simulink model "PP_hinhhoc"  (R2024a)
settings: Solver=ode4  StartTime=0.0  StopTime=10  FixedStep=0.01  RelTol=1e-3
settings Model: Creator=thunguyen  LastModifiedBy=thunguyen

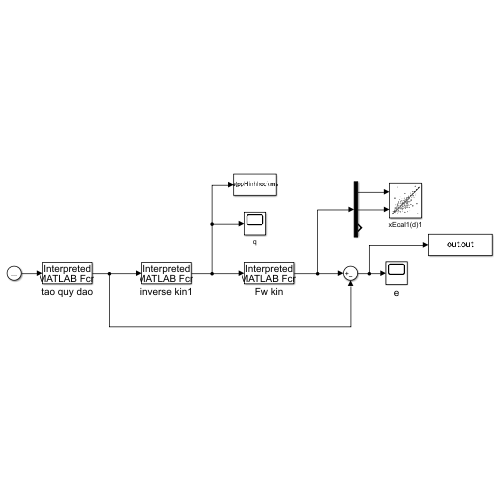
[thumbnail: Simulink's stored preview of the top-level diagram]
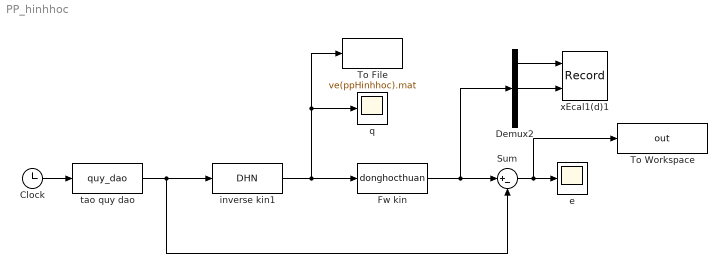
== system PP_hinhhoc ==
  Clock : Clock
  Demux2 : Demux  Outputs=3
  Fw kin : MATLABFcn  MATLABFcn=donghocthuan  OutputDimensions=3  Output1D=off
  Sum : Sum  Inputs=|+-
  To File : ToFile  Filename=ve(ppHinhhoc).mat
  To Workspace : ToWorkspace  VariableName=out  SaveFormat=Timeseries  SampleTime=-1
  e : Scope
  inverse kin1 : MATLABFcn  MATLABFcn=DHN  OutputDimensions=3  Output1D=off
  q : Scope
  tao quy dao : MATLABFcn  MATLABFcn=quy_dao  OutputDimensions=3  Output1D=off
  xEcal1(d)1 : Record  FileSettingsInternal="{\"entries\":[{\"content\":{\"excelSettings\":{\"content\":{},\"type\":\"Streamout.ExcelSettings\"}},\"type\":\"Streamout.FileSettingStorage\",\"uuid\":\"\"}],\"packageUris\":[\"http:\\/\\/schema.mathworks.com\\/mf0\\/streamout_blocks\\/R2020a\"],\"version\":\"1.0\"}"  Layout=[1 1]  SignalsInternal="{\"entries\":[{\"content\":{\"signals\":[{\"content\":{\"blockPath\":[],\"dimensions\":[1],\"domain\":\"\",\"lineColor\":\"#a2142f\",\"lineWidth\":2,\"plots\":[ 1 ],\"port\":1,\"sid\":[\"\"],\"signalID\":1,\"signalName\":\"Demux2:1\"},\"type\":\"RecordBlkView.Signal\",\"uuid\":\"\"},{\"content\":{\"blockPath\":[],\"dimensions\":[1],\"domain\":\"\",\"lineColor\":\"#139fff\",\"lineWidth\":2,\"plots\":[ 1 ],\"port\":2,\"sid\":[\"\"],\"signalID\":2,\"signalName\":\"Demux2:2\"},\"type\":\"RecordBlkView.Signal\",\"uuid\":\"\"}]},\"type\":\"RecordBlkView.InputSignals\",\"uuid\":\"\"}],\"packageUris\":[\"http:\\/\\/schema.mathworks.com\\/mf0\\/streamout_blocks\\/R2020a\"],\"version\":\"1.0\"}"  VisualizationBindings="{\"xyplotplugin\":{\"info\":[{\"series\":[{\"bindingParametersList\":[{\"parameter\":\"X-Axis\",\"signalID\":1,\"signalName\":\"Demux2:1\"},{\"parameter\":\"Y-Axis\",\"signalID\":2,\"signalName\":\"Demux2:2\"}],\"seriesID\":0}],\"subplotID\":1}]}}"  CompatibilityTag=XY
  wires:
  Clock/1 -> tao quy dao/1
  Sum/1 -> To Workspace/1, e/1
  inverse kin1/1 -> To File/1, q/1, Fw kin/1
  tao quy dao/1 -> inverse kin1/1, Sum/2
  Demux2/1 -> xEcal1(d)1/1
  Fw kin/1 -> Demux2/1, Sum/1
  Demux2/2 -> xEcal1(d)1/2
